simulink model "Q2_3_simulink"  (R2022b)
settings: Solver=VariableStepAuto  StartTime=0.0  StopTime=50  RelTol=1e-3
values from neighbouring files (symbols this model uses):
  Km = 39.6*0.001    (= 0.0396)    [Control_prelab_1.m]    (also in preparation_work1.m)
settings Model: Creator=X1  LastModifiedBy=X1

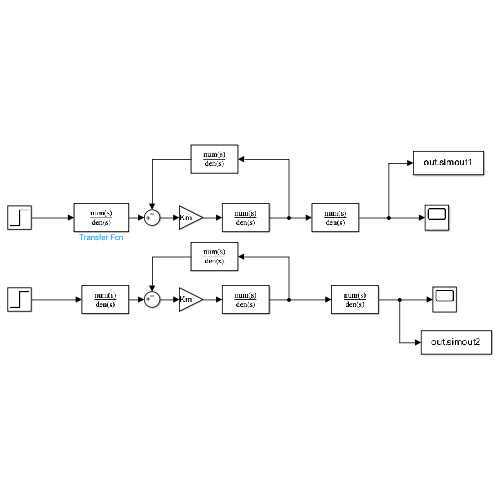
[thumbnail: Simulink's stored preview of the top-level diagram]
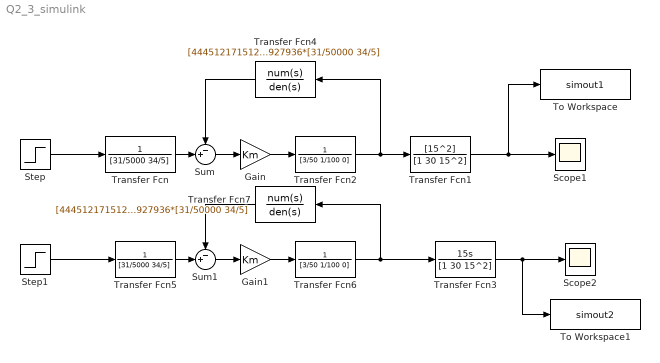
== system Q2_3_simulink ==
  Gain : Gain  Gain=Km
  Gain1 : Gain  Gain=Km
  Scope1 : Scope
  Scope2 : Scope
  Step : Step  Time=0  SampleTime=0
  Step1 : Step  Time=0  SampleTime=0
  Sum : Sum  Inputs=-+|
  Sum1 : Sum  Inputs=-+|
  To Workspace : ToWorkspace  VariableName=simout1  SaveFormat=Timeseries  SampleTime=-1
  To Workspace1 : ToWorkspace  VariableName=simout2  SaveFormat=Timeseries  SampleTime=-1
  Transfer Fcn : TransferFcn  Denominator=[31/5000 34/5]
  Transfer Fcn1 : TransferFcn  Numerator=[15^2]  Denominator=[1 30 15^2]
  Transfer Fcn2 : TransferFcn  Denominator=[3/50 1/100 0]
  Transfer Fcn3 : TransferFcn  Numerator=[15 0]  Denominator=[1 30 15^2]
  Transfer Fcn4 : TransferFcn  Numerator=[4445121715125405 0]  Denominator=72057594037927936*[31/50000 34/5]
  Transfer Fcn5 : TransferFcn  Denominator=[31/5000 34/5]
  Transfer Fcn6 : TransferFcn  Denominator=[3/50 1/100 0]
  Transfer Fcn7 : TransferFcn  Numerator=[4445121715125405 0]  Denominator=72057594037927936*[31/50000 34/5]
  wires:
  Transfer Fcn2/1 -> Transfer Fcn4/1, Transfer Fcn1/1
  Transfer Fcn3/1 -> To Workspace1/1, Scope2/1
  Step/1 -> Transfer Fcn/1
  Gain/1 -> Transfer Fcn2/1
  Transfer Fcn/1 -> Sum/2
  Sum/1 -> Gain/1
  Transfer Fcn4/1 -> Sum/1
  Transfer Fcn1/1 -> To Workspace/1, Scope1/1
  Gain1/1 -> Transfer Fcn6/1
  Transfer Fcn5/1 -> Sum1/2
  Sum1/1 -> Gain1/1
  Transfer Fcn6/1 -> Transfer Fcn3/1, Transfer Fcn7/1
  Transfer Fcn7/1 -> Sum1/1
  Step1/1 -> Transfer Fcn5/1
